simulink model "sf_semantics_hotel_checkin"  (Simulink 7.6)
settings: Solver=FixedStepDiscrete  StartTime=0.0  StopTime=Inf  FixedStep=0.2  RelTol=1e-3
libraries: simulink x4
settings Model: Creator=The MathWorks Inc.
settings DataIOCC: SaveCompleteFinalSimState=on
settings OptimizationCC: InitFltsAndDblsToZero=on
settings DebuggingCC: StrictBusMsg=Warning
settings SFSimCC: SimParseCustomCode=off
settings RTWCC: GenerateReport=on  LaunchReport=on

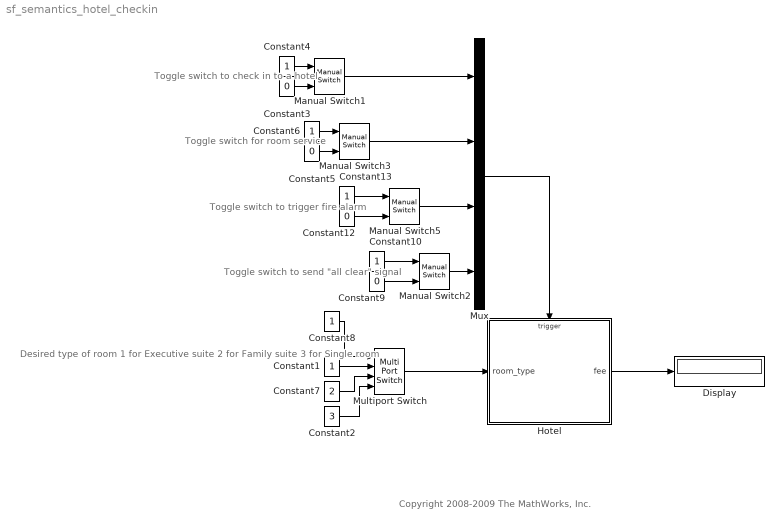
== system sf_semantics_hotel_checkin ==
  note: Desired type of room
      | 1 for Executive suite
      | 2 for Family suite
      | 3 for Single room
  note: Toggle switch to
      | check in to a hotel
  note: Toggle switch
      | for room service
  note: Toggle switch
      | to trigger fire alarm
  note: Toggle switch to
      | send "all clear" signal
  note: Copyright 2008-2009 The MathWorks, Inc.
  Constant{1,4,6,8,10,13} (6 alike) : Constant
  Constant{3,5,9,12} (4 alike) : Constant  Value=0
  Constant2 : Constant  Value=3
  Constant7 : Constant  Value=2
  Display : Display
  Hotel : Stateflow chart  TreatAsAtomicUnit=on
  Manual Switch1 : simulink/Signal Routing/Manual Switch  SystemSampleTime=-1  sw=0  action=0  varsize=off
  Manual Switch2 : simulink/Signal Routing/Manual Switch  SystemSampleTime=-1  sw=1  action=0  varsize=off
  Manual Switch3 : simulink/Signal Routing/Manual Switch  SystemSampleTime=-1  sw=1  action=0  varsize=off
  Manual Switch5 : simulink/Signal Routing/Manual Switch  SystemSampleTime=-1  sw=1  action=0  varsize=off
  Multiport Switch : MultiPortSwitch  zeroidx=off
  Mux : Mux
  wires:
  Constant4/1 -> Manual Switch1/1
  Constant3/1 -> Manual Switch1/2
  Hotel/1(fee) -> Display/1
  Manual Switch1/1 -> Mux/1
  Manual Switch3/1 -> Mux/2
  Mux/1 -> Hotel/Trigger
  Multiport Switch/1 -> Hotel/1(room_type)
  Constant1/1 -> Multiport Switch/2
  Constant2/1 -> Multiport Switch/4
  Constant7/1 -> Multiport Switch/3
  Constant8/1 -> Multiport Switch/1
  Constant6/1 -> Manual Switch3/1
  Constant5/1 -> Manual Switch3/2
  Constant13/1 -> Manual Switch5/1
  Constant12/1 -> Manual Switch5/2
  Manual Switch5/1 -> Mux/3
  Constant10/1 -> Manual Switch2/1
  Constant9/1 -> Manual Switch2/2
  Manual Switch2/1 -> Mux/4

== stateflow chart Hotel ==
  settings: executeAtInitialization=1
  state Check_in
    (history)
    state Front_desk
      exit:
      move_bags = 1;
    state Checked_in
      entry:
      move_bags = 0;
      on room_service:
      service++;
      fee = expenses(service);
      (history)
      state Single_room
      state Executive_suite
        (history)
        state Bedroom
        state Dining_area
        (default) -> Bedroom
        Bedroom -> Dining_area : room_service
        Dining_area -> Bedroom : room_service
      state Family_suite
        state Master_bedroom [parallel]
          settings: executionOrder=1
        state Second_bedroom [parallel]
          settings: executionOrder=2
    (junction 16) -> Single_room : [room_type == 3]  {fee = 500;}
    (default) -> Front_desk
    (junction 17) -> (junction 15) [order 1]
    Front_desk -> (junction 17) : check_in
    (junction 17) -> (junction 16) [order 3]
    (junction 15) -> Executive_suite : [room_type == 1]  {fee = 1500;}
    (junction 17) -> Family_suite [order 2] : [room_type == 2]  {fee = 1000;}
  state Waiting_area
  (default) -> Check_in
  Check_in -> Waiting_area : fire_alarm
  Waiting_area -> Check_in : all_clear
  data: y function_output double; x function_input double; move_bags local double; room_type input double; fee output double; service local double =0
  events: check_in input EITHER_EDGE_EVENT; room_service input EITHER_EDGE_EVENT; fire_alarm input EITHER_EDGE_EVENT; all_clear input EITHER_EDGE_EVENT
  function y = expenses(x):
    | function y = expenses(x)
    | 
    | if (room_type == 1)
    |    y = 1500 + (x*50);    
    | else
    |    if (room_type == 2)
    |       y = 1000 + (x*25);
    |    else 
    |       y = 500 + (x*5);
    |    end
    | end
